simulink model "MotorTestHarness"  (R2024b)
settings: Solver=VariableStepAuto  StartTime=0.0  StopTime=300  RelTol=1e-3
PreLoadFcn:
  | MotorTestHarnessParams;
libraries: fl_lib x24, nesl_utility x10, simulink x5, EmotorLib x1, sdl_lib x1
settings Model: Creator=jjha  LastModifiedBy=jjha
settings OptimizationCC: ReuseModelBlockBuffer=off
settings RTWCC: GPUComputeCapability=3.5

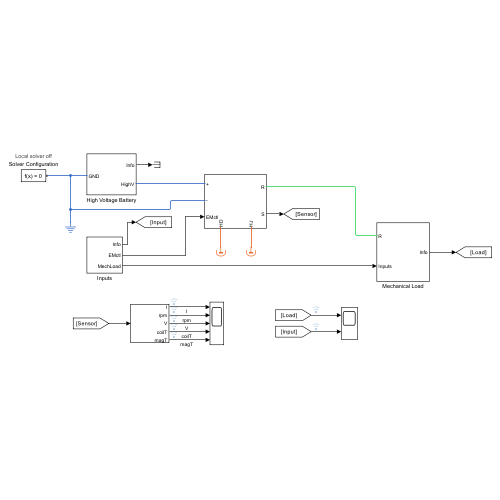
[thumbnail: Simulink's stored preview of the top-level diagram]
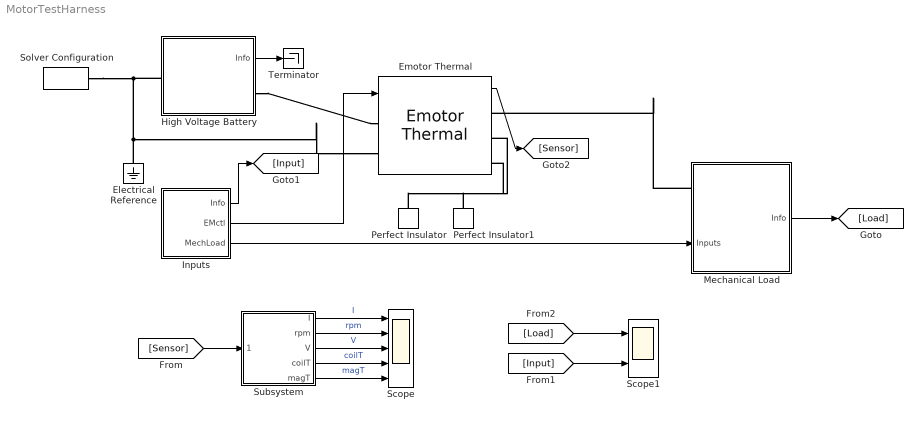
== system MotorTestHarness ==
  Electrical Reference : fl_lib/Electrical/Electrical Elements/Electrical Reference
  Emotor Thermal : EmotorLib/Emotor Thermal  InitTemp=298.15  IronSpHeat=447  CopperSpHeat=385  IronThConductivity=50  GrossToothMass=0.4836  WindingMass=0.4464  max_torque=220  max_power=50000  Tctc=0.002  spMat=[500,10000]  tqMat=[10,200]  lossMat=[0 0;0 0]  StatorBackIronMass=1.997  StatorRootDia=0.1521  stator_od=0.19812  StatorWindingOhArea=0.0538  Bridgemass=0.0698  rotor_od=.12997  rotorStackLength=0.1516  RotorBackIronMass=16.3802  RotorAreaER=0.0265  RotorAreaCyl=0.0619
  High Voltage Battery : Subsystem
  Inputs : Subsystem
  Mechanical Load : Subsystem
      settings: PortSchema="{\"entries\":[{\"content\":{\"sides\":[{\"content\":{\"connectorIds\":[\"LConn1\",\"In1\"]},\"type\":\"ConnectorPlacement.EquallySpacedRectSide\",\"uuid\":\"18221845-08ef-4cf2-b090-320221152030\"},{\"content\":{\"connectorIds\":[\"Out1\"],\"side\":\"RIGHT\"},\"type\":\"ConnectorPlacement.EquallySpacedRectSide\",\"uuid\":\"d5b0548b-74c8-455a-9783-7dc299f3571f\"},{\"content\":{\"connectorIds\":[],\"side\":\"TOP\"},\"type\":\"ConnectorPlacement.EquallySpacedRectSide\",\"uuid\":\"542d8e55-6d7f-4c9a-9fdc-66897ed9f466\"}]},\"type\":\"ConnectorPlacement.EquallySpacedConnector\",\"uuid\":\"3cd4c536-0337-4305-a842-969bfb1fefe3\"}],\"packageUris\":[\"http://schema.mathworks.com/mf0/Connector/R2020b\"],\"version\":\"1.0\"}"
  Perfect Insulator : fl_lib/Thermal/Thermal Elements/Perfect Insulator  T_specify=off  T_priority=None  T=293.15 K  T_nominal_specify=off  T_nominal_value=1  T_nominal_unit=K
  Perfect Insulator1 : fl_lib/Thermal/Thermal Elements/Perfect Insulator  T_specify=off  T_priority=None  T=293.15 K  T_nominal_specify=off  T_nominal_value=1  T_nominal_unit=K
  Scope : Scope  NumInputPorts=5
  Scope1 : Scope  NumInputPorts=2
  Solver Configuration : nesl_utility/Solver Configuration  PhysicalDomain=network_engine_domain  SubClassName=solver  LeftPortType=input  RightPortType=generic  Tones=[]  Harmonics=[]  SimulateNoise=off  Profile=off  UseLocalSampling=off  EnableSwitchedLinearOptims=on  FrequencyDomain=off  UseCCode=off  RelTol=0.001  AbsTol=1e-06  MinStep=1e-09  ToWorkspace=off  RevertToSquareIcSolve=off  NumHomotopyIterations=100  PhasorMode=off  PhasorModeNumHarmonics=1  ConsistencySolver=NEWTON_XTOL_AFTER_FTOL  IndexReductionMethod=DerivativeReplacement  DoDC=off  ResidualTolerance=1e-09  ConsistencyTolSource=GLOBAL  ConsistencyAbsTol=0.001  ConsistencyRelTol=0.001  ConsistencyTolFactor=0.001  UseLocalSolver=off  LocalSolverChoice=NE_BACKWARD_EULER_ADVANCER  ResolveIndetEquations=on  FunctionEvalNumThread=1  LocalSolverSampleTime=0.001  DoFixedCost=off  MaxNonlinIter=3  MaxModeIter=2  ComputeImpulses=off  ImpulseIterations=2  LinearAlgebra=auto  LinearAlgebraNumThread=0  EquationFormulation=NE_TIME_EF  DelaysMemoryBudget=1024  AutomaticFiltering=on  FilteringTimeConstant=0.001  PartitionStorageMethod=AS_NEEDED  PartitionMemoryBudget=1024  PartitionMethod=ROBUST  MultibodyUseLocalSolver=off  MultibodyLocalSolverChoice=ODE1  MultibodyLocalSolverSampleTime=0.001
      settings: AttributesFormatString=Local solver %<UseLocalSolver>
  Subsystem : Subsystem
  Terminator : Terminator
  wires:
  Inputs/3(MechLoad) -> Mechanical Load/1(Inputs)
  Inputs/2(EMctl) -> Emotor Thermal/1
  High Voltage Battery/1(Info) -> Terminator/1
  Inputs/1(Info) -> [Input]
  Mechanical Load/1(Info) -> [Load]
  [Sensor] -> Subsystem/1(" ")
  Subsystem/1(I) -> Scope/1  "I"
  Subsystem/2(rpm) -> Scope/2  "rpm"
  Subsystem/3(V) -> Scope/3  "V"
  Subsystem/4(coilT) -> Scope/4  "coilT"
  Subsystem/5(magT) -> Scope/5  "magT"
  [Input] -> Scope1/2
  [Load] -> Scope1/1
  Emotor Thermal/1 -> [Sensor]
  connections:
  Solver Configuration/RConn1 -- Electrical Reference/LConn1 -- Emotor Thermal/LConn2 -- High Voltage Battery/LConn1
  High Voltage Battery/RConn1 -- Emotor Thermal/LConn1
  Perfect Insulator1/LConn1 -- Emotor Thermal/RConn3
  Perfect Insulator/LConn1 -- Emotor Thermal/RConn2
  Mechanical Load/LConn1 -- Emotor Thermal/RConn1

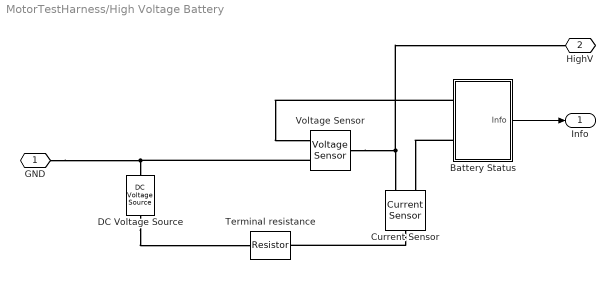
== system MotorTestHarness/High Voltage Battery ==
  Battery Status : Subsystem
  Current Sensor : fl_lib/Electrical/Electrical Sensors/Current Sensor
  DC Voltage Source : fl_lib/Electrical/Electrical Sources/DC Voltage Source  v0=420 V
      settings: AttributesFormatString=%<v0> [%<v0_unit>]
  Terminal resistance : fl_lib/Electrical/Electrical Elements/Resistor  R=0.01 Ohm  i_specify=off  i_priority=High  i=0 A  i_nominal_specify=off  i_nominal_value=1  i_nominal_unit=A  v_specify=off  v_priority=High  v=0 V  v_nominal_specify=off  v_nominal_value=1  v_nominal_unit=V
      settings: AttributesFormatString=%<R> [%<R_unit>]
  Voltage Sensor : fl_lib/Electrical/Electrical Sensors/Voltage Sensor
  GND : PMIOPort  Side=Left
  HighV : PMIOPort  Port=2  Side=Right
  Info : Outport
  wires:
  Battery Status/1(Info) -> Info/1
  connections:
  DC Voltage Source/RConn1 -- GND/RConn1 -- Voltage Sensor/RConn2
  Battery Status/LConn2 -- Current Sensor/RConn1
  Voltage Sensor/LConn1 -- HighV/RConn1 -- Current Sensor/RConn2
  Current Sensor/LConn1 -- Terminal resistance/RConn1
  DC Voltage Source/LConn1 -- Terminal resistance/LConn1
  Battery Status/LConn1 -- Voltage Sensor/RConn1

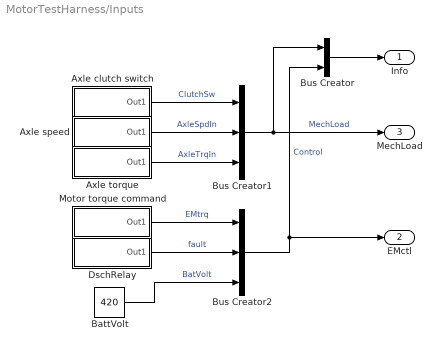
== system MotorTestHarness/Inputs ==
  Axle clutch switch : Subsystem  mask(Piece-Wise Constant Signal){dataPoints=[0 0;1 0]}
      mask prompts: dataPoints "Data points"
      mask help:
      | This block generates a piece-wise constant signal. Data points parameter takes an N-by-2 matrix where each row specifies a constant segment. First column defines the start time of constant segment, and second column specifies the value of it. The value continues until the value of the next segment is defined. The values of the two consecutive rows are connected with a discrete jump.
      |
      | For example, a matrix [0 6; 1 7;2 5] for Data points defines a signal as follows. First row defines a constant segment from t=0 of value 6. Second row defines a point at t=1 of value 7. Third row defines a constant segment from t=2 of value 5. The value makes a discrete jump from one segment to the next.
      mask init:
      | sig = SignalDesigner("PieceWiseConstant");
      | 
      | % Initialization function can access parameter names directly
      | sig.XYData = dataPoints;
      | 
      | update(sig)
      | 
      | SignalSourceBlockCallback.setDataToLookupTableBlock( ...
      |   SignalObject = sig, ...
      |   PathToBlock = [gcb '/1-D Lookup Table']);
      mask DialogControl Control3 Prompt: invisible horizontal spacer 1
      mask DialogControl Control4 Prompt: invisible horizontal spacer 2
      mask DialogControl Control5 Prompt: invisible horizontal spacer 3
      mask DialogControl PlotButton Prompt: Plot
      mask DialogControl PlotButton Callback: SignalSourceBlockCallback.plotPieceWiseConstant(gcb)
      mask Display: disp("Piece-Wise" + newline + "Constant")
  Axle speed : Subsystem  mask(Continuous Multi-Step Signal){dataPoints=[0 1 0], deltaT=10}
      mask prompts: dataPoints "Data points"; deltaT "Interpolation step [s]"
      mask help:
      | This block generates a signal consisting of smoothly connected flat segments. Data points parameter takes an N-by-3 matrix where each row specifies a flat segment. First column and second column define start and end time of the segment, respectively. Third column defines the value of the segment. Second column can also be NaN to define a point value. Flat segments and point values are smoothly interpolated by Akima spline with the specified interpolation step.
      |
      | For example, a matrix [0 1 5; 3 nan 9; 6 8 7] for Data points defines a signal as follows. First row defines a flat segment from t=0 to t=1 of value 5. Second row defines a point at t=3 of value 9. Third row defines a flat segment from t=6 to t=8 of value 7.
      mask init:
      | sig = SignalDesigner("ContinuousMultiStep");
      | 
      | % Initialization function can access parameter names directly
      | sig.XYData = dataPoints;
      | sig.DeltaX = deltaT;
      | 
      | update(sig)
      | 
      | SignalSourceBlockCallback.setDataToLookupTableBlock( ...
      |   SignalObject = sig, ...
      |   PathToBlock = [gcb '/1-D Lookup Table']);
      mask DialogControl Control3 Prompt: horizontal spacer 1
      mask DialogControl Control4 Prompt: horizontal spacer 2
      mask DialogControl Control5 Prompt: horizontal spacer 3
      mask DialogControl PlotButton Prompt: Plot
      mask DialogControl PlotButton Callback: SignalSourceBlockCallback.plotContinuousMultiStep(gcb);
      mask Display: disp("Continuous" + newline + "Multi-Step")
  Axle torque : Subsystem  mask(Continuous Multi-Step Signal){dataPoints=[0 20 0;21 300 -10], deltaT=0.1}
      mask prompts: dataPoints "Data points"; deltaT "Interpolation step [s]"
      mask help:
      | This block generates a signal consisting of smoothly connected flat segments. Data points parameter takes an N-by-3 matrix where each row specifies a flat segment. First column and second column define start and end time of the segment, respectively. Third column defines the value of the segment. Second column can also be NaN to define a point value. Flat segments and point values are smoothly interpolated by Akima spline with the specified interpolation step.
      |
      | For example, a matrix [0 1 5; 3 nan 9; 6 8 7] for Data points defines a signal as follows. First row defines a flat segment from t=0 to t=1 of value 5. Second row defines a point at t=3 of value 9. Third row defines a flat segment from t=6 to t=8 of value 7.
      mask init: same as MotorTestHarness/Inputs/Axle speed
      mask DialogControl Control3 Prompt: horizontal spacer 1
      mask DialogControl Control4 Prompt: horizontal spacer 2
      mask DialogControl Control5 Prompt: horizontal spacer 3
      mask DialogControl PlotButton Prompt: Plot
      mask DialogControl PlotButton Callback: SignalSourceBlockCallback.plotContinuousMultiStep(gcb);
      mask Display: disp("Continuous" + newline + "Multi-Step")
  BattVolt : Constant  Value=420
  Bus Creator : BusCreator  Inputs=2
  Bus Creator1 : BusCreator  Inputs=3
  Bus Creator2 : BusCreator  Inputs=3
  DschRelay : Subsystem  mask(Continuous Multi-Step Signal){dataPoints=[0 50 0;60 200 -2000;250 300 -12000], deltaT=1}
      mask prompts: dataPoints "Data points"; deltaT "Interpolation step [s]"
      mask help:
      | This block generates a signal consisting of smoothly connected flat segments. Data points parameter takes an N-by-3 matrix where each row specifies a flat segment. First column and second column define start and end time of the segment, respectively. Third column defines the value of the segment. Second column can also be NaN to define a point value. Flat segments and point values are smoothly interpolated by Akima spline with the specified interpolation step.
      |
      | For example, a matrix [0 1 5; 3 nan 9; 6 8 7] for Data points defines a signal as follows. First row defines a flat segment from t=0 to t=1 of value 5. Second row defines a point at t=3 of value 9. Third row defines a flat segment from t=6 to t=8 of value 7.
      mask init: same as MotorTestHarness/Inputs/Axle speed
      mask DialogControl Control3 Prompt: horizontal spacer 1
      mask DialogControl Control4 Prompt: horizontal spacer 2
      mask DialogControl Control5 Prompt: horizontal spacer 3
      mask DialogControl PlotButton Prompt: Plot
      mask DialogControl PlotButton Callback: SignalSourceBlockCallback.plotContinuousMultiStep(gcb);
      mask Display: disp("Continuous" + newline + "Multi-Step")
  Motor torque command : Subsystem  mask(Continuous Multi-Step Signal){dataPoints=[0 20 0;60 100 300;105 200 -200;205 300 250], deltaT=0.5}
      mask prompts: dataPoints "Data points"; deltaT "Interpolation step [s]"
      mask help:
      | This block generates a signal consisting of smoothly connected flat segments. Data points parameter takes an N-by-3 matrix where each row specifies a flat segment. First column and second column define start and end time of the segment, respectively. Third column defines the value of the segment. Second column can also be NaN to define a point value. Flat segments and point values are smoothly interpolated by Akima spline with the specified interpolation step.
      |
      | For example, a matrix [0 1 5; 3 nan 9; 6 8 7] for Data points defines a signal as follows. First row defines a flat segment from t=0 to t=1 of value 5. Second row defines a point at t=3 of value 9. Third row defines a flat segment from t=6 to t=8 of value 7.
      mask init: same as MotorTestHarness/Inputs/Axle speed
      mask DialogControl Control3 Prompt: horizontal spacer 1
      mask DialogControl Control4 Prompt: horizontal spacer 2
      mask DialogControl Control5 Prompt: horizontal spacer 3
      mask DialogControl PlotButton Prompt: Plot
      mask DialogControl PlotButton Callback: SignalSourceBlockCallback.plotContinuousMultiStep(gcb);
      mask Display: disp("Continuous" + newline + "Multi-Step")
  Info : Outport
  EMctl : Outport  Port=2
  MechLoad : Outport  Port=3
  wires:
  Bus Creator/1 -> Info/1
  Motor torque command/1(Out1) -> Bus Creator2/1  "EMtrq"
  Axle torque/1(Out1) -> Bus Creator1/3  "AxleTrqIn"
  Axle speed/1(Out1) -> Bus Creator1/2  "AxleSpdIn"
  Axle clutch switch/1(Out1) -> Bus Creator1/1  "ClutchSw"
  Bus Creator1/1 -> Bus Creator/1, MechLoad/1  "MechLoad"
  Bus Creator2/1 -> Bus Creator/2, EMctl/1  "Control"
  DschRelay/1(Out1) -> Bus Creator2/2  "fault"
  BattVolt/1 -> Bus Creator2/3  "BatVolt"

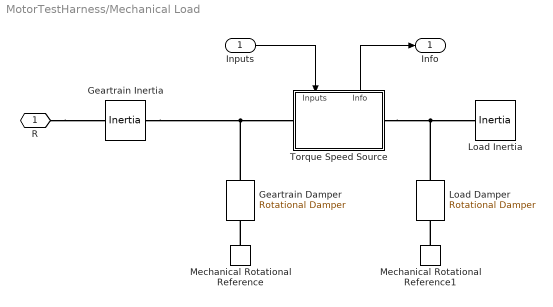
== system MotorTestHarness/Mechanical Load ==
  Inputs : Inport
  Geartrain Damper : fl_lib/Mechanical/Rotational Elements/Rotational Damper  D=0.001 m*N/rpm  w_specify=off  w_priority=None  w=0 rad/s  w_nominal_specify=off  w_nominal_value=1  w_nominal_unit=rad/s  t_specify=off  t_priority=None  t=0 N*m  t_nominal_specify=off  t_nominal_value=1  t_nominal_unit=N*m
      settings: AttributesFormatString=|
      | %<D>
      | %<D_unit>
  Geartrain Inertia : fl_lib/Mechanical/Rotational Elements/Inertia  inertia=1.35 kg*m^2  num_ports=foundation.enum.numPorts2.two  w_specify=on  w_priority=None  w=0 rpm  w_nominal_specify=off  w_nominal_value=1  w_nominal_unit=rad/s  t_specify=off  t_priority=None  t=0 N*m  t_nominal_specify=off  t_nominal_value=1  t_nominal_unit=N*m
      settings: InternalSimscapePortConfiguration="{\"Bottom\":[],\"Left\":[{\"id\":\"I\",\"label\":\"\",\"type\":\"foundation.mechanical.rotational.rotational\"}],\"Right\":[{\"id\":\"J\",\"label\":\"\",\"type\":\"foundation.mechanical.rotational.rotational\"}],\"Top\":[]}"
      settings: AttributesFormatString=|
      | %<inertia> %<inertia_unit>
      | Priority: %<w_priority>
  Load Damper : fl_lib/Mechanical/Rotational Elements/Rotational Damper  D=0.03 N*m/rpm  w_specify=off  w_priority=None  w=0 rad/s  w_nominal_specify=off  w_nominal_value=1  w_nominal_unit=rad/s  t_specify=off  t_priority=None  t=0 N*m  t_nominal_specify=off  t_nominal_value=1  t_nominal_unit=N*m
      settings: AttributesFormatString=|
      | %<D>
      | %<D_unit>
  Load Inertia : fl_lib/Mechanical/Rotational Elements/Inertia  inertia=9 kg*m^2  num_ports=foundation.enum.numPorts2.one  w_specify=off  w_priority=High  w=initial.loadInertiaSpd_rpm rpm  w_nominal_specify=off  w_nominal_value=1  w_nominal_unit=rad/s  t_specify=off  t_priority=None  t=0 N*m  t_nominal_specify=off  t_nominal_value=1  t_nominal_unit=N*m
      settings: AttributesFormatString=|
      | %<inertia> [%<inertia_unit>]
      | %<w> [%<w_unit>]
      | Priority: %<w_priority>
  Mechanical Rotational Reference : fl_lib/Mechanical/Rotational Elements/Mechanical Rotational Reference
  Mechanical Rotational Reference1 : fl_lib/Mechanical/Rotational Elements/Mechanical Rotational Reference
  Torque Speed Source : Subsystem
      settings: PortSchema="{\"entries\":[{\"content\":{\"sides\":[{\"content\":{\"connectorIds\":[\"LConn1\"]},\"type\":\"ConnectorPlacement.EquallySpacedRectSide\",\"uuid\":\"92a06674-aaa2-495f-b380-fd1e5a218eb3\"},{\"content\":{\"connectorIds\":[\"RConn1\"],\"side\":\"RIGHT\"},\"type\":\"ConnectorPlacement.EquallySpacedRectSide\",\"uuid\":\"3e9807eb-b215-4ab1-ac02-6574a58f93c0\"},{\"content\":{\"connectorIds\":[\"In1\",\"Out1\"],\"side\":\"TOP\"},\"type\":\"ConnectorPlacement.EquallySpacedRectSide\",\"uuid\":\"937668c8-63b6-43a7-85c7-81bf7d359316\"}]},\"type\":\"ConnectorPlacement.EquallySpacedConnector\",\"uuid\":\"ba9b6e46-9639-4838-8d50-8636a64d3a24\"}],\"packageUris\":[\"http://schema.mathworks.com/mf0/Connector/R2020b\"],\"version\":\"1.0\"}"
  R : PMIOPort  Side=Left
  Info : Outport
  wires:
  Torque Speed Source/1(Info) -> Info/1
  Inputs/1 -> Torque Speed Source/1(Inputs)
  connections:
  Mechanical Rotational Reference/LConn1 -- Geartrain Damper/RConn1
  Mechanical Rotational Reference1/LConn1 -- Load Damper/RConn1
  R/RConn1 -- Geartrain Inertia/RConn1
  Torque Speed Source/RConn1 -- Load Damper/LConn1 -- Load Inertia/LConn1
  Geartrain Inertia/LConn1 -- Geartrain Damper/LConn1 -- Torque Speed Source/LConn1

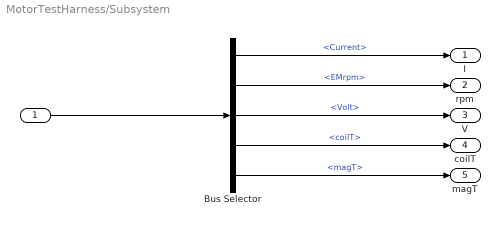
== system MotorTestHarness/Subsystem ==
  " " : Inport
  Bus Selector : BusSelector  OutputSignals=Current,EMrpm,Volt,coilT,magT
  I : Outport
  rpm : Outport  Port=2
  V : Outport  Port=3
  coilT : Outport  Port=4
  magT : Outport  Port=5
  wires:
  " "/1 -> Bus Selector/1
  Bus Selector/2 -> rpm/1  "<EMrpm>"
  Bus Selector/1 -> I/1  "<Current>"
  Bus Selector/3 -> V/1  "<Volt>"
  Bus Selector/4 -> coilT/1  "<coilT>"
  Bus Selector/5 -> magT/1  "<magT>"

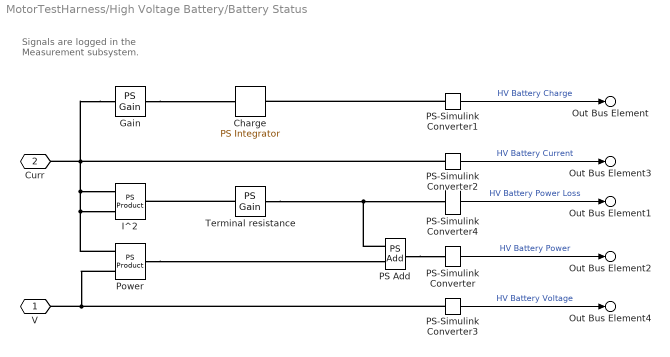
== system MotorTestHarness/High Voltage Battery/Battery Status ==
  note: Signals are logged in
      | the Measurement subsystem.
  Charge : fl_lib/Physical Signals/Linear Operators/PS Integrator  reset_method=foundation.enum.IntegratorResetSpec.None  initial_condition_spec=foundation.enum.IntegratorICSpec.Internal  saturation_spec=foundation.enum.IntegratorSaturationSpec.None  saturation_source_spec=foundation.enum.IntegratorSaturationSourceSpec.Internal  x0=0 A*hr  xu=inf s  xl=-inf s
      settings: AttributesFormatString=%<x0> [%<x0_unit>]
  Gain : fl_lib/Physical Signals/Functions/PS Gain  gain=-1
      settings: AttributesFormatString=%<gain>
  I^2 : fl_lib/Physical Signals/Functions/PS Product
  PS Add : fl_lib/Physical Signals/Functions/PS Add
  PS-Simulink Converter : nesl_utility/PS-Simulink Converter  PhysicalDomain=network_engine_domain  SubClassName=ps_output  LeftPortType=input  RightPortType=output  PseudoPeriodic=off  Frequencies=[]  VectorFormat=1-D array  Unit=kW  AffineConversion=off
  PS-Simulink Converter1 : nesl_utility/PS-Simulink Converter  PhysicalDomain=network_engine_domain  SubClassName=ps_output  LeftPortType=input  RightPortType=output  PseudoPeriodic=off  Frequencies=[]  VectorFormat=1-D array  Unit=A*hr  AffineConversion=off
  PS-Simulink Converter2 : nesl_utility/PS-Simulink Converter  PhysicalDomain=network_engine_domain  SubClassName=ps_output  LeftPortType=input  RightPortType=output  PseudoPeriodic=off  Frequencies=[]  VectorFormat=1-D array  Unit=A  AffineConversion=off
  PS-Simulink Converter3 : nesl_utility/PS-Simulink Converter  PhysicalDomain=network_engine_domain  SubClassName=ps_output  LeftPortType=input  RightPortType=output  PseudoPeriodic=off  Frequencies=[]  VectorFormat=1-D array  Unit=V  AffineConversion=off
  PS-Simulink Converter4 : nesl_utility/PS-Simulink Converter  PhysicalDomain=network_engine_domain  SubClassName=ps_output  LeftPortType=input  RightPortType=output  PseudoPeriodic=off  Frequencies=[]  VectorFormat=1-D array  Unit=W  AffineConversion=off
  Power : fl_lib/Physical Signals/Functions/PS Product
  Terminal resistance : fl_lib/Physical Signals/Functions/PS Gain  gain=0.01 Ohm
      settings: AttributesFormatString=%<gain> [%<gain_unit>]
  V : PMIOPort  Side=Left
  Curr : PMIOPort  Port=2  Side=Left
  Out Bus Element : Outport  PortName=Info  Element=Charge
      settings: AttributesFormatString=%<Unit>
  Out Bus Element3 : Outport  PortName=Info  Element=Current
      settings: AttributesFormatString=%<Unit>
  Out Bus Element1 : Outport  PortName=Info  Element=PowerLoss
      settings: AttributesFormatString=%<Unit>
  Out Bus Element2 : Outport  PortName=Info  Element=Power
      settings: AttributesFormatString=%<Unit>
  Out Bus Element4 : Outport  PortName=Info  Element=Voltage
      settings: AttributesFormatString=%<Unit>
  wires:
  PS-Simulink Converter3/1 -> Out Bus Element4/1  "HV Battery Voltage"
  PS-Simulink Converter2/1 -> Out Bus Element3/1  "HV Battery Current"
  PS-Simulink Converter4/1 -> Out Bus Element1/1  "HV Battery Power Loss"
  PS-Simulink Converter1/1 -> Out Bus Element/1  "HV Battery Charge"
  PS-Simulink Converter/1 -> Out Bus Element2/1  "HV Battery Power"
  connections:
  Power/RConn1 -- PS Add/LConn2
  PS Add/RConn1 -- PS-Simulink Converter/LConn1
  Terminal resistance/LConn1 -- I^2/RConn1
  PS-Simulink Converter1/LConn1 -- Charge/RConn1
  Gain/RConn1 -- Charge/LConn1
  PS Add/LConn1 -- Terminal resistance/RConn1 -- PS-Simulink Converter4/LConn1
  Power/LConn1 -- V/RConn1 -- PS-Simulink Converter3/LConn1
  Gain/LConn1 -- PS-Simulink Converter2/LConn1 -- Curr/RConn1 -- I^2/LConn1 -- Power/LConn2 -- I^2/LConn2

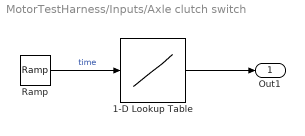
== system MotorTestHarness/Inputs/Axle clutch switch ==
  1-D Lookup Table : Lookup_n-D  NumberOfTableDimensions=1  BreakpointsForDimension1="[0  1]"  Table="[0  0]"  InterpMethod=Flat  InternalRulePriority=Speed  RndMeth=Simplest
  Ramp : simulink/Sources/Ramp  slope=1  start=0  InitialOutput=0
      settings: AttributesFormatString=|
      | Slope: %<slope>
      | Start time: %<start>
      | Initial output: %<InitialOutput>
  Out1 : Outport
  wires:
  Ramp/1 -> 1-D Lookup Table/1  "time"
  1-D Lookup Table/1 -> Out1/1

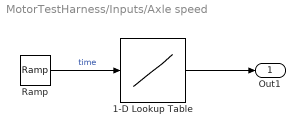
== system MotorTestHarness/Inputs/Axle speed ==
  1-D Lookup Table : Lookup_n-D  NumberOfTableDimensions=1  BreakpointsForDimension1="[0  1]"  Table="[0  0]"  InternalRulePriority=Speed  RndMeth=Simplest
  Ramp : simulink/Sources/Ramp  slope=1  start=0  InitialOutput=0
      settings: AttributesFormatString=|
      | Slope: %<slope>
      | Start time: %<start>
      | Initial output: %<InitialOutput>
  Out1 : Outport
  wires:
  1-D Lookup Table/1 -> Out1/1
  Ramp/1 -> 1-D Lookup Table/1  "time"

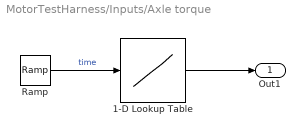
== system MotorTestHarness/Inputs/Axle torque ==
  1-D Lookup Table : Lookup_n-D  NumberOfTableDimensions=1  BreakpointsForDimension1="[0            20          20.1          20.2          20.3          20.4          20.5          20.6          20.7          20.8          20.9            21           300]"  Table="[0            0        -0.28        -1.04        -2.16        -3.52           -5        -6.48        -7.84        -8.96        -9.72          -10          -10]"  InternalRulePriority=Speed  RndMeth=Simplest
  Ramp : simulink/Sources/Ramp  slope=1  start=0  InitialOutput=0
      settings: AttributesFormatString=|
      | Slope: %<slope>
      | Start time: %<start>
      | Initial output: %<InitialOutput>
  Out1 : Outport
  wires:
  Ramp/1 -> 1-D Lookup Table/1  "time"
  1-D Lookup Table/1 -> Out1/1

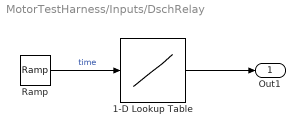
== system MotorTestHarness/Inputs/DschRelay ==
  1-D Lookup Table : Lookup_n-D  NumberOfTableDimensions=1  BreakpointsForDimension1="[0   50   51   52   53   54   55   56   57   58   59   60  200  201  202  203  204  205  206  207  208  209  210  211  212  213  214  215  216  217  218  219  220  221  222  223  224  225  226  227  228  229  230  231  232  233  234  235  236  237  238  239  240  241  242  243  244  245  246  247  248  249  250  300]"  Table="[0               0             -56            -208            -432            -704           -1000           -1296           -1568           -1792           -1944           -2000           -2000        -2011.84        -2046.72        -2103.68        -2181.76           -2280        -2397.44        -2533.12        -2686.08        -2855.36           -3040        -3239.04        -3451.52        -3676.48        -3912.96           -4160        -4416.64        -4681.92        -4954.88        -5234.56           -5520        -5810.24        -6104.32        -6401.28        -6700.16           -7000        -7299.84        -7598.72        -7895.68        -8189.76           -8480        -8765.44        -9045.12        -9318.08        -9583.36           -9840       -10087.04       -10323.52       -10548.48       -10760.96          -10960       -11144.64       -11313.92       -11466.88       -11602.56          -11720       -11818.24       -11896.32       -11953.28       -11988.16          -12000          -12000]"  InternalRulePriority=Speed  RndMeth=Simplest
  Ramp : simulink/Sources/Ramp  slope=1  start=0  InitialOutput=0
      settings: AttributesFormatString=|
      | Slope: %<slope>
      | Start time: %<start>
      | Initial output: %<InitialOutput>
  Out1 : Outport
  wires:
  Ramp/1 -> 1-D Lookup Table/1  "time"
  1-D Lookup Table/1 -> Out1/1

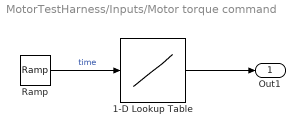
== system MotorTestHarness/Inputs/Motor torque command ==
  1-D Lookup Table : Lookup_n-D  NumberOfTableDimensions=1  BreakpointsForDimension1="[0            20          20.5            21          21.5            22          22.5            23          23.5            24          24.5            25          25.5            26          26.5            27          27.5            28          28.5            29          29.5            30          30.5            31          31.5            32          32.5            33          33.5            34          34.5            35          35.5            36          36.5            37          37.5            38          38.5            39          39.5            40          40.5            41          41.5            42          42.5            43          43.5            44          44.5            45          45.5            46          46.5            47          47.5            48          48.5            49          49.5            50          50.5            51          51.5            52          52.5            53          53.5            54          54.5            55          55.5            56          56.5            57          57.5            58          58.5            59          59.5            60           100         100.5           101         101.5           102         102.5           103         103.5           104         104.5           105           200         200.5           201         201.5           202         202.5           203         203.5           204         204.5           205           300]"  Table="[0             0     0.1394531      0.553125      1.233984         2.175      3.369141      4.809375      6.488672           8.4      10.53633      12.89062      15.45586        18.225      21.19102      24.34687      27.68555          31.2       34.8832      38.72813      42.72773        46.875      51.16289      55.58438      60.13242          64.8      69.58008      74.46563      79.44961        84.525      89.68477      94.92188      100.2293         105.6       111.027      116.5031      122.0215       127.575      133.1566      138.7594      144.3762           150      155.6238      161.2406      166.8434       172.425      177.9785      183.4969       188.973         194.4      199.7707      205.0781      210.3152       215.475      220.5504      225.5344      230.4199         235.2      239.8676      244.4156      248.8371       253.125      257.2723      261.2719      265.1168         268.8      272.3145      275.6531       278.809       281.775      284.5441      287.1094      289.4637         291.6      293.5113      295.1906      296.6309       297.825       298.766      299.4469      299.8605           300           300           286           248           192           124            50           -24           -92          -148          -186          -200          -200        -187.4        -153.2        -102.8         -41.6            25          91.6         152.8         203.2         237.4           250           250]"  InternalRulePriority=Speed  RndMeth=Simplest
  Ramp : simulink/Sources/Ramp  slope=1  start=0  InitialOutput=0
      settings: AttributesFormatString=|
      | Slope: %<slope>
      | Start time: %<start>
      | Initial output: %<InitialOutput>
  Out1 : Outport
  wires:
  1-D Lookup Table/1 -> Out1/1
  Ramp/1 -> 1-D Lookup Table/1  "time"

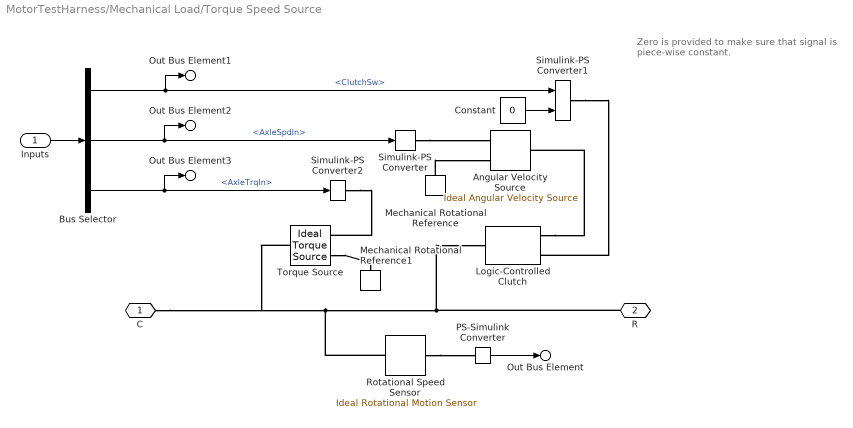
== system MotorTestHarness/Mechanical Load/Torque Speed Source ==
  note: Zero is provided to make sure
      | that signal is piece-wise constant.
  Inputs : Inport
  Angular Velocity Source : fl_lib/Mechanical/Mechanical Sources/Ideal Angular Velocity Source
  Bus Selector : BusSelector  OutputSignals=ClutchSw,AxleSpdIn,AxleTrqIn
  Constant : Constant  Value=0
  Logic-Controlled Clutch : sdl_lib/Clutches/Logic-Controlled Clutch  transition_model=sdl.enum.transitionModel.instant  transition_time_constant=0.1 s  t_friction=5000 N*m  t_locked=5000 N*m  w_tol=0.1 rpm  initial_state_locked=sdl.enum.initial_lock.unlocked
      settings: InternalSimscapePortConfiguration="{\"Bottom\":[],\"Left\":[{\"id\":\"E\",\"label\":\"E\",\"type\":\"input\"},{\"id\":\"B\",\"label\":\"B\",\"type\":\"foundation.mechanical.rotational.rotational\"}],\"Right\":[{\"id\":\"F\",\"label\":\"F\",\"type\":\"foundation.mechanical.rotational.rotational\"}],\"Top\":[]}"
  Mechanical Rotational Reference : fl_lib/Mechanical/Rotational Elements/Mechanical Rotational Reference
  Mechanical Rotational Reference1 : fl_lib/Mechanical/Rotational Elements/Mechanical Rotational Reference
  PS-Simulink Converter : nesl_utility/PS-Simulink Converter  PhysicalDomain=network_engine_domain  SubClassName=ps_output  LeftPortType=input  RightPortType=output  PseudoPeriodic=off  Frequencies=[]  VectorFormat=inherit  Unit=rpm  AffineConversion=off
  Rotational Speed Sensor : fl_lib/Mechanical/Mechanical Sensors/Ideal Rotational Motion Sensor  reference=foundation.enum.MeasurementReference.absolute  acceleration_port=false  velocity_port=true  position_port=false  wrap_angle=simscape.enum.onoff.off  offset=0 rad
      settings: InternalSimscapePortConfiguration="{\"Bottom\":[],\"Left\":[{\"id\":\"R\",\"label\":\"R\",\"type\":\"foundation.mechanical.rotational.rotational\"}],\"Right\":[{\"id\":\"W\",\"label\":\"W\",\"type\":\"output\"}],\"Top\":[]}"
  Simulink-PS Converter : nesl_utility/Simulink-PS Converter  PhysicalDomain=network_engine_domain  SubClassName=ps_input  LeftPortType=input  RightPortType=output  PseudoPeriodic=off  Frequencies=[]  NoiseDistribution=none  NoiseParameters=[]  Unit=rpm  AffineConversion=off  FilteringAndDerivatives=filter  SimscapeFilterOrder=1  InputFilterTimeConstant=0.001  UdotUserProvided=1
  Simulink-PS Converter1 : nesl_utility/Simulink-PS Converter  PhysicalDomain=network_engine_domain  SubClassName=ps_input  LeftPortType=input  RightPortType=output  PseudoPeriodic=off  Frequencies=[]  NoiseDistribution=none  NoiseParameters=[]  Unit=1  AffineConversion=off  FilteringAndDerivatives=provide  SimscapeFilterOrder=1  InputFilterTimeConstant=0.001  UdotUserProvided=1
      settings: AttributesFormatString=|
      | %<Unit>
      | Derivative: %<FilteringAndDerivatives>
  Simulink-PS Converter2 : nesl_utility/Simulink-PS Converter  PhysicalDomain=network_engine_domain  SubClassName=ps_input  LeftPortType=input  RightPortType=output  PseudoPeriodic=off  Frequencies=[]  NoiseDistribution=none  NoiseParameters=[]  Unit=N*m  AffineConversion=off  FilteringAndDerivatives=filter  SimscapeFilterOrder=1  InputFilterTimeConstant=0.001  UdotUserProvided=1
  Torque Source : fl_lib/Mechanical/Mechanical Sources/Ideal Torque Source
  C : PMIOPort  Side=Left
  R : PMIOPort  Port=2  Side=Right
  Out Bus Element : Outport  PortName=Info  Element=AxleSpd
  Out Bus Element1 : Outport  PortName=Info  Element=AxleClutchSw
  Out Bus Element2 : Outport  PortName=Info  Element=AxleSpdIn
  Out Bus Element3 : Outport  PortName=Info  Element=AxleTrqIn
  wires:
  Inputs/1 -> Bus Selector/1
  Bus Selector/1 -> Simulink-PS Converter1/1, Out Bus Element1/1  "<ClutchSw>"
  Bus Selector/2 -> Simulink-PS Converter/1, Out Bus Element2/1  "<AxleSpdIn>"
  Bus Selector/3 -> Out Bus Element3/1, Simulink-PS Converter2/1  "<AxleTrqIn>"
  PS-Simulink Converter/1 -> Out Bus Element/1
  Constant/1 -> Simulink-PS Converter1/2
  connections:
  Simulink-PS Converter/RConn1 -- Angular Velocity Source/RConn1
  Mechanical Rotational Reference/LConn1 -- Angular Velocity Source/RConn2
  Logic-Controlled Clutch/LConn2 -- Angular Velocity Source/LConn1
  Simulink-PS Converter1/RConn1 -- Logic-Controlled Clutch/LConn1
  Rotational Speed Sensor/LConn1 -- R/RConn1 -- Logic-Controlled Clutch/RConn1 -- C/RConn1 -- Torque Source/LConn1
  Rotational Speed Sensor/RConn1 -- PS-Simulink Converter/LConn1
  Simulink-PS Converter2/RConn1 -- Torque Source/RConn1
  Torque Source/RConn2 -- Mechanical Rotational Reference1/LConn1
